simulink model "serial_i2c_PCF8474Read"  (R2015a)
settings: Solver=FixedStepDiscrete  SolverMode=SingleTasking  StartTime=0.0  StopTime=10.0  FixedStep=1e-3  RelTol=1e-3
libraries: mbed_lib x7, simulink x3
settings Model: Creator=oh  LastModifiedBy=oh
settings OptimizationCC: OptimizeModelRefInitCode=on  LifeSpan=1
settings HardwareCC: ProdLargestAtomicInteger=Long  ProdLargestAtomicFloat=Double  ProdEndianess=LittleEndian  ProdHWDeviceType=ARM Compatible->ARM Cortex
settings RTWCC: SystemTargetFile=mbed.tlc  TemplateMakefile=mbed.tmf  Description=Mbed Target (Embedded Target)  TargetLang=C++
settings CodeAppCC: IgnoreCustomStorageClasses=off
settings STFCustomTargetCC: CombineOutputUpdateFcns=on  SupportContinuousTime=off  SupportVariableSizeSignals=off  SystemTargetFile=mbed.tlc
settings ERTTargetCC: SupportContinuousTime=off  SupportVariableSizeSignals=off  ERTCustomFileTemplate=mbed_file_process.tlc

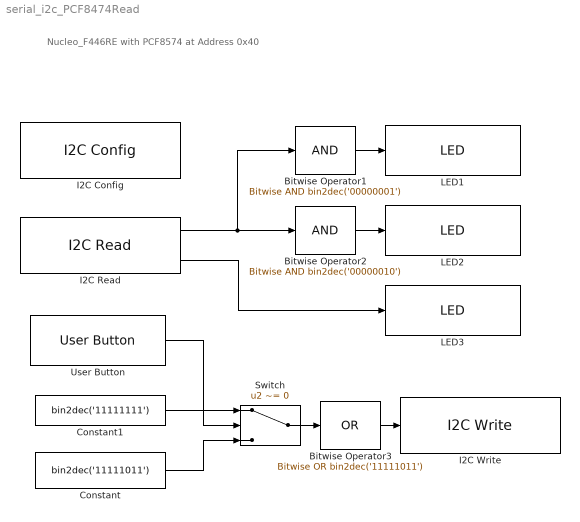
== system serial_i2c_PCF8474Read ==
  note: Nucleo_F446RE with PCF8574 at Address 0x40
  Bitwise Operator1 : simulink/Logic and Bit Operations/Bitwise Operator  logicop=AND  UseBitMask=on  BitMask=bin2dec('00000001')  BitMaskRealWorld=Stored Integer
  Bitwise Operator2 : simulink/Logic and Bit Operations/Bitwise Operator  logicop=AND  UseBitMask=on  BitMask=bin2dec('00000010')  BitMaskRealWorld=Stored Integer
  Bitwise Operator3 : simulink/Logic and Bit Operations/Bitwise Operator  logicop=OR  UseBitMask=on  BitMask=bin2dec('11111011')  BitMaskRealWorld=Stored Integer
  Constant : Constant  Value=bin2dec('11111011')  OutDataTypeStr=uint8
  Constant1 : Constant  Value=bin2dec('11111111')  OutDataTypeStr=uint8
  I2C Config : mbed_lib/Serial/I2C/I2C Config  Priority=0  I2CPort=1  Freq=100000  SDAPortName=B  SDAPinNumber=9  SCLPortName=B  SCLPinNumber=8
  I2C Read : mbed_lib/Serial/I2C/I2C Read  I2cPort=1  AddressFlag=off  SlaveAddress=64  ByteCountFlag=off  NumBytes=1  Repeated=off  AckOut=on  SampleTime=0.1
  I2C Write : mbed_lib/Serial/I2C/I2C Write  I2cPort=1  AddressFlag=off  SlaveAddress=64  ByteCountFlag=off  Repeated=off  AckOut=off  SampleTime=-1
  LED1 : mbed_lib/GPIO/LED  nLED=1  SampleTime=-1
  LED2 : mbed_lib/GPIO/LED  nLED=2  SampleTime=-1
  LED3 : mbed_lib/GPIO/LED  nLED=3  SampleTime=-1
  Switch : Switch  Criteria=u2 ~= 0
  User Button : mbed_lib/GPIO/User Button  SampleTime=0.1
  wires:
  Bitwise Operator1/1 -> LED1/1
  Bitwise Operator2/1 -> LED2/1
  Switch/1 -> Bitwise Operator3/1
  User Button/1 -> Switch/2
  Bitwise Operator3/1 -> I2C Write/1
  Constant1/1 -> Switch/1
  Constant/1 -> Switch/3
  I2C Read/1 -> Bitwise Operator1/1, Bitwise Operator2/1
  I2C Read/2 -> LED3/1
